simulink model "ex16"  (Simulink 6.0)
settings: Solver=ode45  StartTime=0.0  StopTime=10  MaxStep=0.001  RelTol=1e-3
undefined symbols (not defined in the file or in its folder): Fs, get, magnitude
libraries: dspstat3 x2, dspsnks4 x2, commanapbnd2 x1, commrandsrc2 x1
settings Model: LastModifiedBy=lxy

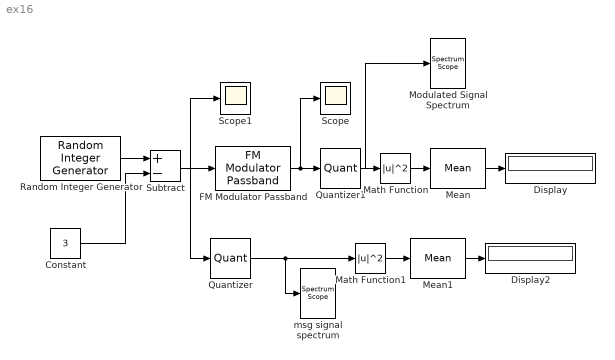
== system ex16 ==
  Constant : Constant  Value=3
  Display : Display
  Display2 : Display
  FM Modulator Passband : commanapbnd2/FM Modulator Passband  Fc=250  Ph=0  HzPerV=50  ts=0.001  td=Inf
  Math Function : Math  Operator=magnitude^2  SaturateOnIntegerOverflow=on
  Math Function1 : Math  Operator=magnitude^2  SaturateOnIntegerOverflow=on
  Mean : dspstat3/Mean  DialogController=dspDDGCreate  DialogControllerArgs=DataTag0  run=on  reset_popup=None  roundingMode=Floor  overflowMode=off
  Mean1 : dspstat3/Mean  DialogController=dspDDGCreate  DialogControllerArgs=DataTag1  run=on  reset_popup=None  roundingMode=Floor  overflowMode=off
  "Modulated Signal Spectrum " : dspsnks4/Spectrum Scope  ScopeProperties=on  Domain=Frequency  HorizSpan=1  UseBuffer=on  BufferSize=512  Overlap=256  inpFftLenInherit=on  FFTlength=256  numAvg=2  DisplayProperties=off  AxisGrid=on  Memory=off  FrameNumber=on  AxisLegend=off  AxisZoom=off  OpenScopeAtSimStart=on  OpenScopeImmediately=off  FigPos=get(0,'defaultfigureposition')  AxisProperties=off  XUnits=Hertz  XRange=[-Fs/2...Fs/2]  InheritXIncr=on  XIncr=1.0  XLabel=Samples  YUnits=dB  YLabel=Magnitude, dB  LineProperties=off
      settings: YMin=-50  YMax=50
  Quantizer : Quantizer  QuantizationInterval=0.001  LinearizeAsGain=off  SampleTime=0.001
  Quantizer1 : Quantizer  QuantizationInterval=0.001  LinearizeAsGain=off  SampleTime=0.001
  Random Integer Generator : commrandsrc2/Random Integer Generator  mul=7  seed=1234  Ts=1/10  frameBased=off  sampPerFrame=1  orient=off
  Scope : Scope
  Scope1 : Scope
      settings: YMin=-4  YMax=4
  Subtract : Sum  Inputs=+-  OutScaling=2^-10
  msg signal spectrum : dspsnks4/Spectrum Scope  ScopeProperties=on  Domain=Frequency  HorizSpan=1  UseBuffer=on  BufferSize=512  Overlap=256  inpFftLenInherit=on  FFTlength=512  numAvg=2  DisplayProperties=off  AxisGrid=on  Memory=off  FrameNumber=on  AxisLegend=off  AxisZoom=off  OpenScopeAtSimStart=on  OpenScopeImmediately=off  FigPos=get(0,'defaultfigureposition')  AxisProperties=off  XUnits=Hertz  XRange=[-Fs/2...Fs/2]  InheritXIncr=on  XIncr=1.0  XLabel=Samples  YUnits=dB  YLabel=Magnitude, dB  LineProperties=off
      settings: YMin=-30  YMax=30
  wires:
  Quantizer1/1 -> "Modulated Signal Spectrum "/1, Math Function/1
  Random Integer Generator/1 -> Subtract/1
  Constant/1 -> Subtract/2
  Subtract/1 -> Quantizer/1, Scope1/1, FM Modulator Passband/1
  Quantizer/1 -> msg signal spectrum/1, Math Function1/1
  Mean/1 -> Display/1
  Math Function/1 -> Mean/1
  Math Function1/1 -> Mean1/1
  Mean1/1 -> Display2/1
  FM Modulator Passband/1 -> Scope/1, Quantizer1/1
